simulink model "Dynamic_FFT"  (R2021a)
settings: Solver=VariableStepAuto  StartTime=0.0  StopTime=10*frame_size  RelTol=1e-3
PostLoadFcn:
  | header_size = 4; % For single and int32 data types
InitFcn:
  | header_size = 4; % For single and int32 data types
model workspace (MAT data in the model file):
  FFT_len = 2048
  frame_size = 2048
  max_fft_size = 1024
undefined symbols (not defined in the file): magnitude, S, vsva2197, xcvc1902
libraries: dspstat3 x2, dspmtrx3 x2, aieDSP x1, simulink x1, vmcUtilities x1, dspsrcs4 x1, aieUtilities x1
settings Model: Creator=ravidapu  LastModifiedBy=abehbood
settings SolverCC: AlgebraicLoopSolver=TrustRegion

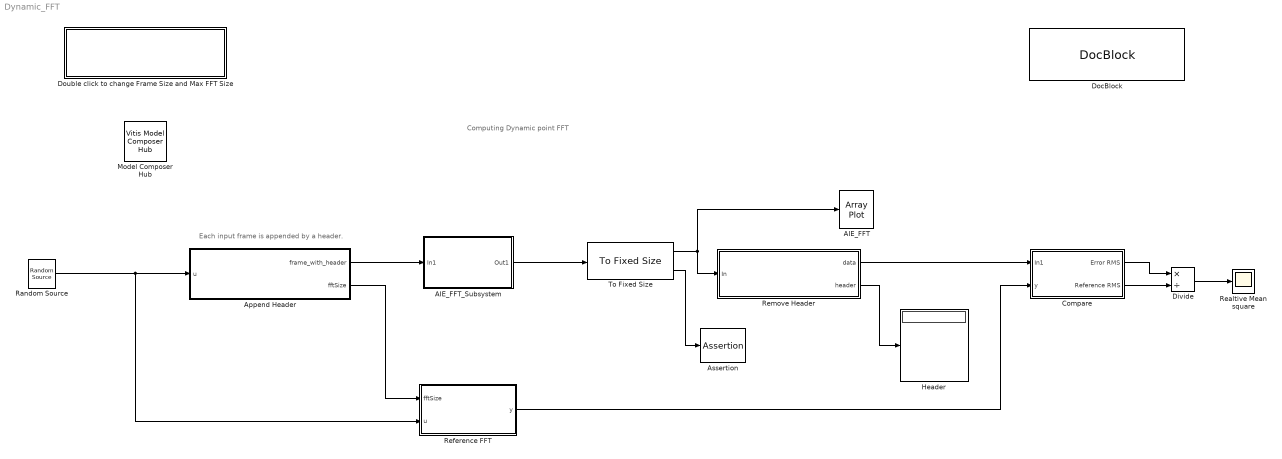
== system Dynamic_FFT ==
  note: Each input frame is appended by a header.
  note: Computing Dynamic point FFT
  AIE_FFT : ArrayPlot  WindowPosition=[880.000000,470.000000,800.000000,500.000000,]  ShowLegend=on  DefaultConfigurationName=dsp.scopes.ArrayPlotBlockSpecification
  AIE_FFT_Subsystem : Subsystem
  Append Header : MATLAB Function  TreatAsAtomicUnit=on  mask{fftSizeInput=[128 512 1024]}
      mask prompts: fftSizeInput "FFT Size"
      mask help:
      | This block appends a header to each incoming frame. The FFT Size parameter specifies an array of power of twos. These should be equal or smaller than the maximum size FFT specified for the Dynamic Point FFT block.
      |
      | As an example, if the FFT Size parameter is [128, 512, 1024] and the input size to this block is 1024, the Dynamic Point FFT block will take a 128 point FFT of the first 128 samples of the first input frame (discarding other samples), a 512 point FFT of the first 512 samples of the second input frame (discarding other samples), and a 1024 point FFT of the third input frame and all the subsequent input frames.
  Assertion : Assertion
  Compare : Subsystem
  Divide : Product  Inputs=*/
  DocBlock : simulink/Model-Wide Utilities/DocBlock  DocumentType=Text  mask(DocBlock){}
      content=|
      | ///////////////////////////////////////////////////////////////////////////
      | // Copyright 2021 Xilinx
      | //
      | // Licensed under the Apache License, Version 2.0 (the "License");
      | // you may not use this file except in compliance with the License.
      | // You may obtain a copy of the License at
      | //
      | // http://www.apache.org/licenses/LICENSE-2.0
      | //
      | // Unless required by applicable law or agreed to in writing, software
      | // distributed under the License is distributed on an "AS IS" BASIS,
      | // WITHOUT WARRANTIES OR CONDITIONS OF ANY KIND, either express or implied.
      | // See the License for the specific language governing permissions and
      | // limitations under the License.
      | ///////////////////////////////////////////////////////////////////////////
      mask Display:
      | xmcDrawBlockIcon();
      | disp(['{\fontsize{10pt}(c) Copyright 2022' ' Xilinx, Inc.}\newline \newline '],'texmode','on');
      | disp('{\fontsize{10pt}Licensed under the Apache License 2.0}','texmode','on');
      | disp('\newline \newline \newline{\fontsize{10pt}Double Click for Copyright Notice}','texmode','on');
  Double click to change Frame Size and Max FFT Size : Subsystem  mask{max_fft_size=1024, frame_size=2048}
      mask prompts: max_fft_size "Max FFT Size"; frame_size "Frame Size"
      mask help: Set the FFT length
      mask TypeOptions max_fft_size: 128 | 256 | 512 | 1024 | 2048 | 4096
      mask Callback max_fft_size:
      | max_fft_size = str2double(get_param(gcb,'max_fft_size'));
      | hws = get_param(bdroot, 'modelworkspace');
      | hws.assignin('max_fft_size', max_fft_size);
      mask Callback frame_size:
      | frame_size = str2double(get_param(gcb,'frame_size'));
      | hws = get_param(bdroot, 'modelworkspace');
      | hws.assignin('frame_size', frame_size);
      mask Display:
      | max_fft_size = get_param(gcb,'max_fft_size');
      | frame_size = get_param(gcb,'frame_size');
      | 
      | disp(['\fontsize{18}Max FFT Size = ' max_fft_size newline 'Frame Size = ' frame_size], 'texmode', 'on');
  Header : Display
  Model Composer Hub : vmcUtilities/Vitis Model Composer Hub  Tag=genX  CodeGeneration=off  SubsystemName=AIE_FFT_Subsystem  TargetDirectory=./code  ExportType=AI Engines  IpVendor=xilinx.com  IpLibrary=hls  IpVersion=1.0  IpHWLanguage=Verilog  AieCompilerOptions={}  CreateTestbench=on  TestbenchStackSize=10  RunAieSim=on  AieSimTimeout=50000  RunAieSimProfiling=off  LaunchVitisAnalyzer=off  PlotOutput=off  RunX86Sim=off  X86SimTimeout=10  GenHwImage=off  PlatformType=Not Specified  HwSystemType=Baremetal  HwValidationTarget=hw  ProjDevice=xcvc1902-vsva2197-2MP-e-S  ProjDevicePart=xcvc1902-vsva2197-2MP-e-S  SamplePeriod=-1  ClockFrequency=200  DataPathParallelism=1  xilinxfamily=Kintex7  part=xc7k325t  speed=-3  package=fbg676  directory=./netlist  testbench=off  incr_netlist=off  synthesis_tool=Vivado  clock_wrapper=Clock Enables  dbl_ovrd=According to Block Masks  dcm_input_clock_period=10  sysclk_period=10  simulink_period=1  eval_field=0
  Random Source : dspsrcs4/Random Source  SrcType=Gaussian  NormMethod=Ziggurat  CltLength=12  MinVal=0  MaxVal=1  MeanVal=0  VarVal=1  RepMode=Not repeatable  rawSeed=1  IsInherit=off  SampMode=Discrete  SampTime=1  SampFrame=frame_size  DataType=Single  OutComplex=Complex  OutputFrames=off
  Realtive Mean square : Scope
  Reference FFT : MATLAB Function  TreatAsAtomicUnit=on
  Remove Header : Subsystem
  To Fixed Size : aieUtilities/To Fixed Size  OutputSize=Inherit: Same as input  CopyMethod=Buffer samples to form output  HasStatusOutput=on
  wires:
  Divide/1 -> Realtive Mean square/1
  Compare/1(Error RMS) -> Divide/1
  Compare/2(Reference RMS) -> Divide/2
  AIE_FFT_Subsystem/1(Out1) -> To Fixed Size/1
  Append Header/1(frame_with_header) -> AIE_FFT_Subsystem/1(In1)
  Append Header/2(fftSize) -> Reference FFT/1(fftSize)
  Reference FFT/1(y) -> Compare/2(y)
  Random Source/1 -> Reference FFT/2(u), Append Header/1(u)
  Remove Header/1(data) -> Compare/1(In1)
  Remove Header/2(header) -> Header/1
  To Fixed Size/1 -> AIE_FFT/1, Remove Header/1(In)
  To Fixed Size/2 -> Assertion/1

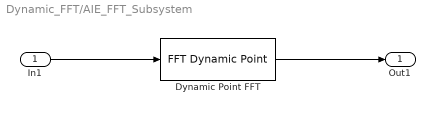
== system Dynamic_FFT/AIE_FFT_Subsystem ==
  In1 : Inport
  Dynamic Point FFT : aieDSP/FFT Dynamic Point  data_type=cfloat  point_size=max_fft_size  input_window_size=frame_size  shift_val=0  input_sampling_rate=200  use_casc_length=on  casc_length=1  spec=meta_data_hl_dyn_pt_fft.json
  Out1 : Outport
  wires:
  In1/1 -> Dynamic Point FFT/1
  Dynamic Point FFT/1 -> Out1/1

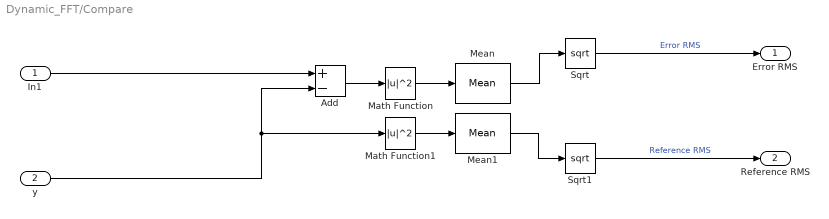
== system Dynamic_FFT/Compare ==
  In1 : Inport
  y : Inport  Port=2
  Add : Sum  Inputs=+-
  Math Function : Math  Operator=magnitude^2  SaturateOnIntegerOverflow=on
  Math Function1 : Math  Operator=magnitude^2  SaturateOnIntegerOverflow=on
  Mean : dspstat3/Mean  run=off  InputProcessing=Columns as channels (frame based)  reset_popup=None  directionMode=Entire input  dimension=1  roiEnable=off  roiType=Rectangles  roiPortion=Entire ROI  roiOutput=Individual statistics for each ROI  roiFlag=off  roundingMode=Floor  overflowMode=off  outputDataTypeStr=Inherit: Same as accumulator  outputMin=[]  outputMax=[]  outputLastDataTypeStr=Inherit: Same as accumulator
  Mean1 : dspstat3/Mean  run=off  InputProcessing=Columns as channels (frame based)  reset_popup=None  directionMode=Entire input  dimension=1  roiEnable=off  roiType=Rectangles  roiPortion=Entire ROI  roiOutput=Individual statistics for each ROI  roiFlag=off  roundingMode=Floor  overflowMode=off  outputDataTypeStr=Inherit: Same as accumulator  outputMin=[]  outputMax=[]  outputLastDataTypeStr=Inherit: Same as accumulator
  Sqrt : Sqrt  SaturateOnIntegerOverflow=on
  Sqrt1 : Sqrt  SaturateOnIntegerOverflow=on
  Error RMS : Outport
  Reference RMS : Outport  Port=2
  wires:
  Math Function1/1 -> Mean1/1
  Sqrt1/1 -> Reference RMS/1  "Reference RMS"
  Math Function/1 -> Mean/1
  Sqrt/1 -> Error RMS/1  "Error RMS"
  Add/1 -> Math Function/1
  y/1 -> Math Function1/1, Add/2
  Mean1/1 -> Sqrt1/1
  In1/1 -> Add/1
  Mean/1 -> Sqrt/1

== system Dynamic_FFT/Double click to change Frame Size and Max FFT Size ==

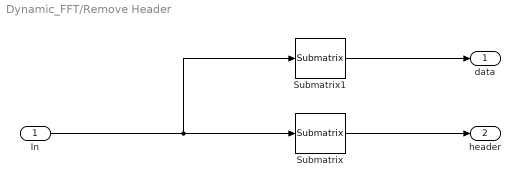
== system Dynamic_FFT/Remove Header ==
  In : Inport
  Submatrix : dspmtrx3/Submatrix  RowSpan=Range of rows  RowStartMode=Index  RowStartIndex=1  RowEndMode=Index  RowEndIndex=4  ColSpan=All columns  ColStartMode=Index  ColStartIndex=1  ColEndMode=Index  ColEndIndex=8
  Submatrix1 : dspmtrx3/Submatrix  RowSpan=Range of rows  RowStartMode=Index  RowStartIndex=5  RowEndMode=Last  RowEndIndex=8  ColSpan=All columns  ColStartMode=Index  ColStartIndex=9  ColEndMode=Last  ColEndIndex=8
  data : Outport
  header : Outport  Port=2
  wires:
  Submatrix1/1 -> data/1
  In/1 -> Submatrix/1, Submatrix1/1
  Submatrix/1 -> header/1

== matlab function Dynamic_FFT/Reference FFT ==
  data: fftSize input; u input; y output; frame_size parameter; max_fft_size parameter
function y = fcn(fftSize, u, frame_size, max_fft_size)

out = complex(zeros(frame_size,1));

for i = 0:frame_size/max_fft_size-1
    frame_fft = fft(double(u(i*max_fft_size+1:(i+1)*max_fft_size)),fftSize);
    out(i*max_fft_size+1:(i+1)*max_fft_size) = [frame_fft; zeros(max_fft_size - fftSize,1)];
end

y = out(1:frame_size);

== matlab function Dynamic_FFT/Append Header ==
  data: u input; frame_with_header output; fftSizeInput parameter; fftSize output size=1
function [frame_with_header, fftSize] = fcn(u, fftSizeInput)

persistent inputFrameNum

if isempty(inputFrameNum)
    inputFrameNum = 1;    
end

headerValueSize = 4; % for int32 and Single data types.  
headerValue = zeros(headerValueSize,1);

% fftSize must be an array of power of twos that are smaller than input size

if any( fftSizeInput > length(u))
    error('fft sizes should be smaller or equal to the block input size.')
end

if ~all(log2(fftSizeInput) == round(log2(fftSizeInput)))
    error('fft sizes must be powers of two.')
end


% 0 for ifft, 1 for ifft
fftDir = 1; 

powerOf2 = log2(fftSizeInput(inputFrameNum)); 

% NOTE: For int16 the header is 8 samples and is in the form of [fftDir powerOf2 0 0 0 0 0 0];

if isa(u,'int32') || isa(u,'single')
    headerValue(:,1) = [fftDir powerOf2 0 0]';
else
    error('While Dynamic FFT block also supports input of type int16, this block only supports input data type of int32 or single.')
end

fftSize = fftSizeInput(inputFrameNum);

% Cap inputFrameNum
if inputFrameNum < length(fftSizeInput)
    inputFrameNum = inputFrameNum + 1;
end

frame_with_header = [headerValue(1:headerValueSize,1); u];
